simulink model "s_VI_operational_InvD_contr_14b"  (Simulink 8.4)
settings: Solver=ode45  SolverMode=SingleTasking  StartTime=0.0  StopTime=5  RelTol=1e-3
values from neighbouring files (symbols this model uses):
  Kd = 50    [m_IV_run_inverse_dynamics_operational.m]
  Kp = 500    [m_IV_run_inverse_dynamics_operational.m]
settings Model: Creator=a_bad  LastModifiedBy=a_bad  CovMetricSettings=dwe  CovHtmlReporting=off  covSaveCumulativeToWorkspaceVar=off  CovSaveSingleToWorkspaceVar=off  CovExternalEMLEnable=on  CovSFcnEnable=on
settings DataIOCC: LimitDataPoints=off  SaveFormat=StructureWithTime  SignalLoggingSaveFormat=Dataset
settings OptimizationCC: ExpressionDepthLimit=128
settings DebuggingCC: AlgebraicLoopMsg=none  UnderspecifiedInitializationDetection=Simplified  MergeDetectMultiDrivingBlocksExec=error  SolverPrmCheckMsg=none  FcnCallInpInsideContextMsg=EnableAllAsError  FrameProcessingCompatibilityMsg=error  StateNameClashWarn=none  SFUnexpectedBacktrackingDiag=error  SFNoUnconditionalDefaultTransitionDiag=error
settings HardwareCC: ProdBitPerPointer=64  ProdLargestAtomicFloat=Float  ProdIntDivRoundTo=Zero  ProdEndianess=LittleEndian  ProdHWDeviceType=Specified
settings ModelReferenceCC: PropagateSignalLabelsOutOfModel=on
settings GRTTargetCC: TargetLangStandard=C99 (ISO)  GeneratePreprocessorConditionals=Use local settings  CombineOutputUpdateFcns=on  GRTInterface=off

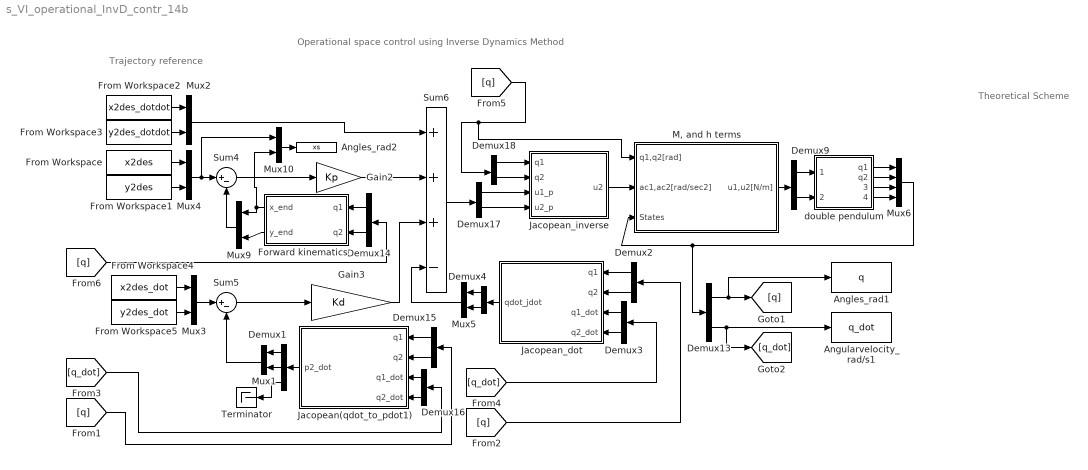
== system s_VI_operational_InvD_contr_14b ==
  note: Theoretical Scheme
  note: Operational space control using Inverse Dynamics Method
  note: Trajectory
      | reference
  Angles_rad1 : ToWorkspace  VariableName=q  SaveFormat=Timeseries  SampleTime=-1
  Angles_rad2 : ToWorkspace  VariableName=xs  SaveFormat=Timeseries  SampleTime=-1
  Angularvelocity_rad/s1 : ToWorkspace  VariableName=q_dot  SaveFormat=Timeseries  SampleTime=-1
  Demux1 : Demux  Outputs=3
  Demux{2..4,9,13..18} (10 alike) : Demux  Outputs=2
  Forward kinematics : MATLAB Function  TreatAsAtomicUnit=on
      settings: PermitHierarchicalResolution=ParametersOnly
  From Workspace : FromWorkspace  VariableName=x2des  SampleTime=0
  From Workspace1 : FromWorkspace  VariableName=y2des  SampleTime=0
  From Workspace2 : FromWorkspace  VariableName=x2des_dotdot  SampleTime=0
  From Workspace3 : FromWorkspace  VariableName=y2des_dotdot  SampleTime=0
  From Workspace4 : FromWorkspace  VariableName=x2des_dot  SampleTime=0
  From Workspace5 : FromWorkspace  VariableName=y2des_dot  SampleTime=0
  Gain2 : Gain  Gain=Kp
  Gain3 : Gain  Gain=Kd
  Jacopean(qdot_to_pdot1) : MATLAB Function  TreatAsAtomicUnit=on
      settings: PermitHierarchicalResolution=ParametersOnly
  Jacopean_dot : MATLAB Function  TreatAsAtomicUnit=on
      settings: PermitHierarchicalResolution=ParametersOnly
  "Jacopean_inverse " : MATLAB Function  TreatAsAtomicUnit=on
      settings: PermitHierarchicalResolution=ParametersOnly
  "M, and h terms" : Subsystem
  Mux{1..5,9..10} (7 alike) : Mux  Inputs=2
  Mux6 : Mux
  Sum4 : Sum  Inputs=|+-
  Sum5 : Sum  Inputs=|+-
  Sum6 : Sum  Inputs=+++-
  Terminator : Terminator
  "double pendulum " : Subsystem
      mask Display: image('294px-Double-Pendulum.svg.png');
  wires:
  Mux6/1 -> Demux13/1, "M, and h terms"/3(States)
  "double pendulum "/3("q1_dot ") -> Mux6/3
  "double pendulum "/4(q2_dot) -> Mux6/4
  "double pendulum "/2("q2  ") -> Mux6/2
  "double pendulum "/1(q1) -> Mux6/1
  Demux9/1 -> "double pendulum "/1(Tau1)
  Demux13/2 -> [q_dot], Angularvelocity_rad/s1/1
  Demux13/1 -> [q], Angles_rad1/1
  Demux9/2 -> "double pendulum "/2("Tau2 ")
  Demux14/1 -> Forward kinematics/1(q1)
  Demux14/2 -> Forward kinematics/2(q2)
  Forward kinematics/2(y_end) -> Mux9/2
  Demux15/1 -> Jacopean(qdot_to_pdot1)/1(q1)
  Demux15/2 -> Jacopean(qdot_to_pdot1)/2(q2)
  Demux16/1 -> Jacopean(qdot_to_pdot1)/3(q1_dot)
  Demux16/2 -> Jacopean(qdot_to_pdot1)/4(q2_dot)
  Sum4/1 -> Gain2/1
  Sum5/1 -> Gain3/1
  Gain2/1 -> Sum6/2
  Gain3/1 -> Sum6/3
  Demux17/1 -> "Jacopean_inverse "/3(u1_p)
  Demux17/2 -> "Jacopean_inverse "/4(u2_p)
  [q] -> Demux18/1, "M, and h terms"/1(q1,q2[rad])
  Demux18/2 -> "Jacopean_inverse "/2(q2)
  Demux18/1 -> "Jacopean_inverse "/1(q1)
  Mux1/1 -> Sum5/2
  Jacopean(qdot_to_pdot1)/1(p2_dot) -> Demux1/1
  Demux1/2 -> Mux1/2
  Demux1/1 -> Mux1/1
  Mux4/1 -> Mux10/1, Sum4/1
  From Workspace1/1 -> Mux4/2
  From Workspace/1 -> Mux4/1
  Demux1/3 -> Terminator/1
  Sum6/1 -> Demux17/1
  Mux3/1 -> Sum5/1
  Mux2/1 -> Sum6/1
  From Workspace2/1 -> Mux2/1
  From Workspace3/1 -> Mux2/2
  From Workspace5/1 -> Mux3/2
  From Workspace4/1 -> Mux3/1
  [q] -> Demux15/1
  [q_dot] -> Demux16/1
  [q] -> Demux14/1
  Mux9/1 -> Sum4/2
  "M, and h terms"/1(u1,u2[N/m]) -> Demux9/1
  "Jacopean_inverse "/1(u2) -> "M, and h terms"/2(ac1,ac2[rad/sec2])
  Mux5/1 -> Sum6/4
  Demux4/1 -> Mux5/1
  Demux2/1 -> Jacopean_dot/1(q1)
  [q] -> Demux2/1
  Demux2/2 -> Jacopean_dot/2(q2)
  Demux3/1 -> Jacopean_dot/3(q1_dot)
  Demux3/2 -> Jacopean_dot/4(q2_dot)
  [q_dot] -> Demux3/1
  Demux4/2 -> Mux5/2
  Jacopean_dot/1(qdot_jdot) -> Demux4/1
  Mux10/1 -> Angles_rad2/1
  Forward kinematics/1(x_end) -> Mux10/2, Mux9/1

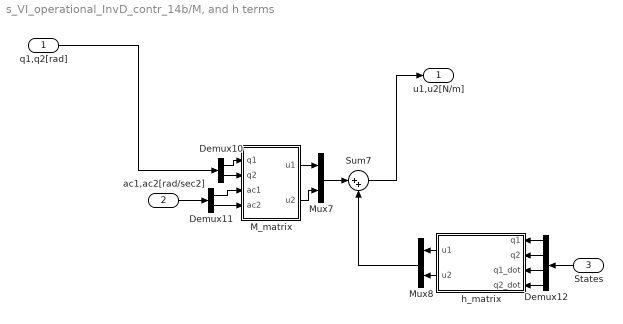
== system s_VI_operational_InvD_contr_14b/M, and h terms ==
  q1,q2[rad] : Inport
  ac1,ac2[rad/sec2] : Inport  Port=2
  States : Inport  Port=3
  Demux10 : Demux  Outputs=2
  Demux11 : Demux  Outputs=2
  Demux12 : Demux
  "M_matrix " : MATLAB Function  TreatAsAtomicUnit=on
      settings: PermitHierarchicalResolution=ParametersOnly
  Mux7 : Mux  Inputs=2
  Mux8 : Mux  Inputs=2
  Sum7 : Sum  Inputs=|++
  "h_matrix " : MATLAB Function  TreatAsAtomicUnit=on
      settings: PermitHierarchicalResolution=ParametersOnly
  u1,u2[N/m] : Outport
  wires:
  Demux12/1 -> "h_matrix "/1(q1)
  Demux12/3 -> "h_matrix "/3(q1_dot)
  Mux7/1 -> Sum7/1
  Demux12/4 -> "h_matrix "/4(q2_dot)
  Demux12/2 -> "h_matrix "/2(q2)
  "h_matrix "/1(u1) -> Mux8/1
  Demux10/2 -> "M_matrix "/2(q2)
  Demux11/2 -> "M_matrix "/4(ac2)
  "h_matrix "/2(u2) -> Mux8/2
  "M_matrix "/1(u1) -> Mux7/1
  Demux10/1 -> "M_matrix "/1(q1)
  "M_matrix "/2(u2) -> Mux7/2
  q1,q2[rad]/1 -> Demux10/1
  Mux8/1 -> Sum7/2
  Demux11/1 -> "M_matrix "/3(ac1)
  ac1,ac2[rad/sec2]/1 -> Demux11/1
  States/1 -> Demux12/1
  Sum7/1 -> u1,u2[N/m]/1

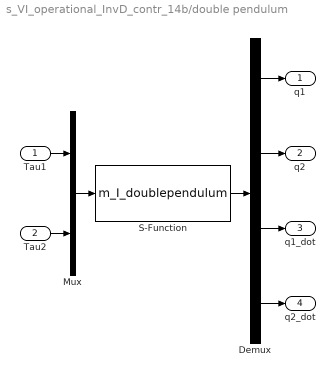
== system s_VI_operational_InvD_contr_14b/double pendulum  ==
  Tau1 : Inport
  "Tau2 " : Inport  Port=2
  Demux : Demux
  Mux : Mux  Inputs=2
  S-Function : S-Function  FunctionName=m_I_doublependulum  Parameters=pi/4 -pi/2 0 0  SFunctionDeploymentMode=off  EnableBusSupport=off
  q1 : Outport
  "q2  " : Outport  Port=2
  "q1_dot " : Outport  Port=3
  q2_dot : Outport  Port=4
  wires:
  Mux/1 -> S-Function/1
  S-Function/1 -> Demux/1
  Tau1/1 -> Mux/1
  "Tau2 "/1 -> Mux/2
  Demux/4 -> q2_dot/1
  Demux/3 -> "q1_dot "/1
  Demux/2 -> "q2  "/1
  Demux/1 -> q1/1

== matlab function Jacopean_dot ==
  data: q1 input double; q2 input double; q1_dot input double; q2_dot input double; qdot_jdot output double
function qdot_jdot  = fcn(q1,q2,q1_dot,q2_dot)

L1=1;L2=1;
% A=[-L1*sin(q1)           0;
%     L1*cos(q1)           0;
%     1                    0]
% B=[-L1*sin(q1)-L2*sin(q1+q2)        -L2*sin(q1+q2);
%     L1*cos(q1)+L2*cos(q1+q2)         L2*cos(q1+q2);
%     1                                1              ];
% p1_dot=A*[q1_dot;q2_dot]
B=[-L1*cos(q1)*q1_dot-L2*cos(q1+q2)*(q1_dot+q2_dot) -L2*cos(q1+q2)*(q1_dot+q2_dot);
   -L1*sin(q1)*q1_dot-L2*sin(q1+q2)*(q1_dot+q2_dot) -L2*sin(q1+q2)*(q1_dot+q2_dot)];
qdot_jdot=B*[q1_dot;q2_dot];

== matlab function M, and h terms/M_matrix  ==
  data: q1 input double; q2 input double; ac1 input double; u1 output double; ac2 input double; u2 output double
function [u1,u2] = fcn(q1,q2,ac1,ac2)
Grav=10;     %%Gravity acceleration constant
M=1;       
L1=1;
L2=1;
Gz=1;
beta=20;
Ts=0.01;    %%sampling time
G1=M*(L1^2+L2^2)+Gz;
G2=M*L2^2+Gz;
H11=G1+2*M*L1*L2*cos(q2);   H12=G2+  M*L1*L2*cos(q2);
H21=G2+  M*L1*L2*cos(q2);   H22=G2;

u1= H11*ac1+H12*ac2;
u2= H21*ac1+H22*ac2;

== matlab function M, and h terms/h_matrix  ==
  data: q1 input double; u1 output double; q2 input double; q1_dot input double; q2_dot input double; u2 output double
function [u1,u2] = fcn(q1,q2,q1_dot,q2_dot)
Grav=10;     %%Gravity acceleration constant
M=1;       
L1=1;
L2=1;
Gz=1;
beta=20;
G1=M*(L1^2+L2^2)+Gz;
G2=M*L2^2+Gz;
C11=-2*M*L1*L2*sin(q2)*q2_dot;  C12=-M*L1*L2*cos(q2)*q2_dot;
C21=M*L1*L2*sin(q2)*q1_dot;     C22=0;
g1=M*Grav*(L1*cos(q1)+L2*cos(q1+q2));    g2=M*Grav*L2*cos(q1+q2);
u1=[C11 C12]*[q1_dot;q2_dot]+g1+[beta 0]*[q1_dot;q2_dot];
u2=[C21 C22]*[q1_dot;q2_dot]+g2+[0 beta]*[q1_dot;q2_dot];

== matlab function Forward kinematics ==
  data: q1 input double; x_end output double; q2 input double; y_end output double
function [x_end,y_end] = fcn(q1,q2)

L1=1;L2=1;

x = [L1*cos(q1),  L1*cos(q1)+L2*cos(q1+q2)];
y = [L1*sin(q1),  L1*sin(q1)+L2*sin(q1+q2)];
x_end=x(2);
y_end=y(2);

== matlab function Jacopean(qdot_to_pdot1) ==
  data: q1 input double; q2 input double; q1_dot input double; q2_dot input double; p2_dot output double
function p2_dot  = fcn(q1,q2,q1_dot,q2_dot)

L1=1;L2=1;
A=[-L1*sin(q1)           0;
    L1*cos(q1)           0;
    1                    0];
B=[-L1*sin(q1)-L2*sin(q1+q2)        -L2*sin(q1+q2);
    L1*cos(q1)+L2*cos(q1+q2)         L2*cos(q1+q2);
    1                                1              ];
p1_dot=A*[q1_dot;q2_dot];
p2_dot=B*[q1_dot;q2_dot];

== matlab function Jacopean_inverse  ==
  data: q1 input double; q2 input double; u1_p input double; u2_p input double; u2 output double
function u2  = fcn(q1,q2,u1_p,u2_p)

L1=1;L2=1;
A=[-L1*sin(q1)           0;
    L1*cos(q1)           0;
  ];

B=[-L1*sin(q1)-L2*sin(q1+q2)        -L2*sin(q1+q2);
    L1*cos(q1)+L2*cos(q1+q2)         L2*cos(q1+q2);
   ];

u1=A*[u1_p;u2_p];
u2=inv(B)*[u1_p;u2_p];
